simulink model "simulator"  (R2018b)
settings: Solver=FixedStepAuto  StartTime=0.0  StopTime=simulation_time  FixedStep=sample_time  RelTol=1e-12
values from neighbouring files (symbols this model uses):
  c_1 = 0.000416568624689888    (= 0.00041656862469)    [Parameters.m]    (also in Parameters2.m)
  c_2 = 0.341159914008612    (= 0.341159914009)    [Parameters.m]    (also in Parameters2.m)
  final_step_value = 3    [Parameters.m]    (also in Parameters2.m = input('Final step value (ex. 3 [bar]): '))
  initial_step_value = 0    [Parameters.m]    (also in Parameters2.m = input('Initial step value (ex. 0 [bar]): '))
  k_i = input('New ki: ')    [Main.m]    (also in Parameters.m = 3; Parameters2.m = input('Ki (ex. 3): '))
  model_initial_condition = 0    [Parameters.m]    (also in Parameters2.m = input('Model initial condition (ex. 0): '))
  output_when_on = 78    [Parameters.m]    (also in Parameters2.m)
  PI_initial_condition = 0    [Parameters.m]    (also in Parameters2.m = input('PI initial condition (ex. 0): '))
  step_time = simulation_time/2    (= 2500)    [Parameters.m]    (also in Parameters2.m = input('Step time (ex. 2500 [s]): '))
  switch_on_point = 1    [Parameters.m]    (also in Parameters2.m)
  time_delay = 10    [Parameters.m]    (also in Parameters2.m = input('Time delay (ex. 10 [s]): '))
settings Model: Creator=paoloesposito  LastModifiedBy=alessandrosebastianelli
settings SolverCC: ZeroCrossAlgorithm=Adaptive
settings DebuggingCC: MaxConsecutiveZCsMsg=none  LibraryContextMissingDiagnostic=none
settings SFSimCC: SimUseLocalCustomCode=off
settings RTWCC: RTWUseLocalCustomCode=off

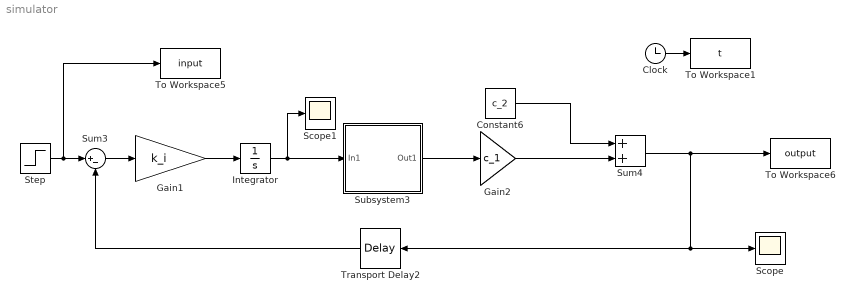
== system simulator ==
  Clock : Clock
  Constant6 : Constant  Value=c_2
  Gain1 : Gain  Gain=k_i
  Gain2 : Gain  Gain=c_1
  Integrator : Integrator  InitialCondition=PI_initial_condition
  Scope : Scope
  Scope1 : Scope
  Step : Step  Time=step_time  Before=initial_step_value  After=final_step_value
  Subsystem3 : Subsystem
  Sum3 : Sum  Inputs=|+-
  Sum4 : Sum
  To Workspace1 : ToWorkspace  VariableName=t  SampleTime=-1
  To Workspace5 : ToWorkspace  VariableName=input  SampleTime=-1
  To Workspace6 : ToWorkspace  VariableName=output  SampleTime=-1
  Transport Delay2 : TransportDelay  DelayTime=time_delay  BufferSize=21504
  wires:
  Clock/1 -> To Workspace1/1
  Gain1/1 -> Integrator/1
  Transport Delay2/1 -> Sum3/2
  Sum3/1 -> Gain1/1
  Integrator/1 -> Scope1/1, Subsystem3/1(In1)
  Step/1 -> To Workspace5/1, Sum3/1
  Subsystem3/1(Out1) -> Gain2/1
  Constant6/1 -> Sum4/1
  Gain2/1 -> Sum4/2
  Sum4/1 -> Scope/1, Transport Delay2/1, To Workspace6/1

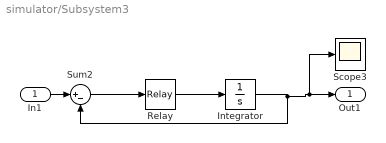
== system simulator/Subsystem3 ==
  In1 : Inport
  Integrator : Integrator  InitialCondition=model_initial_condition
  Relay : Relay  OnSwitchValue=switch_on_point  OffSwitchValue=-switch_on_point  OnOutputValue=output_when_on  OffOutputValue=-output_when_on
  Scope3 : Scope
  Sum2 : Sum  Inputs=|+-
  Out1 : Outport
  wires:
  In1/1 -> Sum2/1
  Relay/1 -> Integrator/1
  Integrator/1 -> Scope3/1, Out1/1, Sum2/2
  Sum2/1 -> Relay/1
